simulink model "sldemo_bpcheck"  (Simulink 6.0)
settings: Solver=ode45  StartTime=0.0  StopTime=10.0  RelTol=1e-3
undefined symbols (not defined in the file or in its folder): membrane
libraries: simulink x9
settings Model: Creator=The MathWorks Inc.  LastModifiedBy=batserve  ExtModeAutoUpdateStatusClock=off
settings DataIOCC: SignalLoggingName=sigsOut
settings OptimizationCC: BooleanDataType=off
settings DebuggingCC: CheckExecutionContextPreStartOutputMsg=on  CheckExecutionContextRuntimeOutputMsg=on  SolverPrmCheckMsg=none
settings HardwareCC: TargetUnknown=on

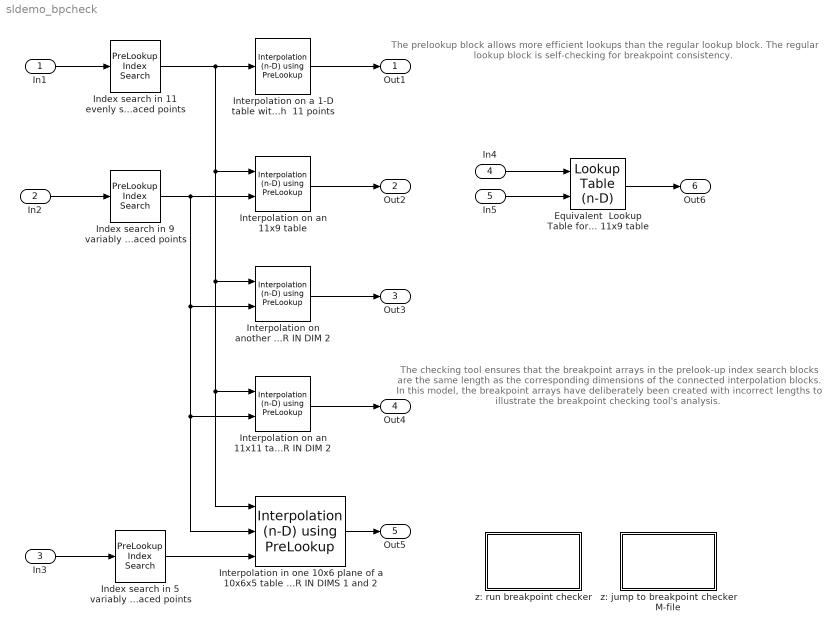
== system sldemo_bpcheck ==
  note: The checking tool ensures that
      | the breakpoint arrays in the
      | prelook-up index search blocks
      | are the same length as the
      | corresponding dimensions of the
      | connected interpolation blocks.
      |
      | In this model, the breakpoint arrays
      | have deliberately been created with
      |  incorrect lengths to illustrate the
      | breakpoint checking tool's analysis.
  note: The prelookup block allows  more
      | efficient lookups than the regular lookup
      | block.  The regular lookup block is
      | self-checking for breakpoint consistency.
  In1 : Inport  Port=1  LatchInput=off
  In2 : Inport  Port=2  LatchInput=off
  In3 : Inport  Port=3  LatchInput=off
  In4 : Inport  Port=4  LatchInput=off
  In5 : Inport  Port=5  LatchInput=off
  Equivalent  Lookup Table for Interpolation on an 11x9 table : simulink/Lookup Tables/Lookup Table (n-D)  numDimsPopupSelect=2  bp1=[0:10:100]  bp2=[ 0.5, 1, 3, 5, 15, 45, 95, 96, 97 ]  bp3=[1:3]  bp4=[1:3]  bpcell={ [1:3], [1:3] }  explicitNumDims=2  searchMode=Binary Search  cacheBpFlag=off  vectorInputFlag=off  tableData=reshape([1:99], [11,9])  interpMethod=Linear  extrapMethod=Linear  rangeErrorMode=None
  Index search in 11 evenly spaced points : simulink/Lookup Tables/PreLookup Index Search  bpData=[0:10:100]  searchMode=Evenly Spaced Points  cacheBpFlag=off  outputFlag=off  IndexDataType=uint32  extrapMode=Linear Extrapolation  rangeErrorMode=None
  Index search in 5 variably spaced points : simulink/Lookup Tables/PreLookup Index Search  bpData=[-100, 125, 150, 200, 500]  searchMode=Linear Search  cacheBpFlag=on  outputFlag=on  IndexDataType=uint32  extrapMode=Clip to Range  rangeErrorMode=Warning
  Index search in 9 variably spaced points : simulink/Lookup Tables/PreLookup Index Search  bpData=[ 0.5, 1, 3, 5, 15, 45, 95, 96, 97 ]  searchMode=Binary Search  cacheBpFlag=on  outputFlag=off  IndexDataType=uint32  extrapMode=Linear Extrapolation  rangeErrorMode=None
  Interpolation in one 10x6 plane of a 10x6x5 table ERROR IN DIMS 1 and 2 : simulink/Lookup Tables/Interpolation (n-D) using PreLookup  numDimsPopupSelect=3  explicitNumDims=2  table=reshape([1:300], [10,6,5])  interpMethod=Linear  extrapMethod=None - Clip  rangeErrorMode=None  NumSelectionDims=1
  Interpolation on a 1-D table with  11 points : simulink/Lookup Tables/Interpolation (n-D) using PreLookup  numDimsPopupSelect=1  explicitNumDims=2  table=[1:11].*[1:11]  interpMethod=Linear  extrapMethod=None - Clip  rangeErrorMode=None  NumSelectionDims=0
  Interpolation on an 11x11 table ERROR IN DIM 2 : simulink/Lookup Tables/Interpolation (n-D) using PreLookup  numDimsPopupSelect=2  explicitNumDims=2  table=sqrt([0:10]'*[0:10])  interpMethod=Linear  extrapMethod=Linear  rangeErrorMode=None  NumSelectionDims=0
  Interpolation on an 11x9 table : simulink/Lookup Tables/Interpolation (n-D) using PreLookup  numDimsPopupSelect=2  explicitNumDims=2  table=reshape([1:99], [11,9])  interpMethod=Linear  extrapMethod=None - Clip  rangeErrorMode=None  NumSelectionDims=0
  Interpolation on another 11x11 table ERROR IN DIM 2 : simulink/Lookup Tables/Interpolation (n-D) using PreLookup  numDimsPopupSelect=2  explicitNumDims=2  table=membrane(1,5,9,9)  interpMethod=Linear  extrapMethod=Linear  rangeErrorMode=None  NumSelectionDims=0
  z: jump to breakpoint checker M-file : Subsystem  PropExecContextAcrossSSBoundary=on
      settings: OpenFcn=edit slcheckprelookups.m
      mask Type: Demo
      mask Display: disp('View\nBreakpoint\nChecker')
  z: run breakpoint checker : Subsystem  PropExecContextAcrossSSBoundary=on
      settings: OpenFcn=evalin('base','preblks = slcheckprelookups(''sldemo_bpcheck''), commandwindow')
      mask Type: Demo
      mask Display: disp('Run\nBreakpoint\nChecker')
  Out1 : Outport
  Out2 : Outport  Port=2
  Out3 : Outport  Port=3
  Out4 : Outport  Port=4
  Out5 : Outport  Port=5
  Out6 : Outport  Port=6
  wires:
  Index search in 11 evenly spaced points/1 -> Interpolation in one 10x6 plane of a 10x6x5 table ERROR IN DIMS 1 and 2/1, Interpolation on an 11x11 table ERROR IN DIM 2/1, Interpolation on another 11x11 table ERROR IN DIM 2/1, Interpolation on an 11x9 table/1, Interpolation on a 1-D table with  11 points/1
  In1/1 -> Index search in 11 evenly spaced points/1
  In2/1 -> Index search in 9 variably spaced points/1
  Index search in 9 variably spaced points/1 -> Interpolation in one 10x6 plane of a 10x6x5 table ERROR IN DIMS 1 and 2/2, Interpolation on an 11x11 table ERROR IN DIM 2/2, Interpolation on another 11x11 table ERROR IN DIM 2/2, Interpolation on an 11x9 table/2
  In3/1 -> Index search in 5 variably spaced points/1
  Index search in 5 variably spaced points/1 -> Interpolation in one 10x6 plane of a 10x6x5 table ERROR IN DIMS 1 and 2/3
  Interpolation on an 11x9 table/1 -> Out2/1
  Interpolation on another 11x11 table ERROR IN DIM 2/1 -> Out3/1
  Interpolation in one 10x6 plane of a 10x6x5 table ERROR IN DIMS 1 and 2/1 -> Out5/1
  Interpolation on a 1-D table with  11 points/1 -> Out1/1
  Interpolation on an 11x11 table ERROR IN DIM 2/1 -> Out4/1
  In4/1 -> Equivalent  Lookup Table for Interpolation on an 11x9 table/1
  In5/1 -> Equivalent  Lookup Table for Interpolation on an 11x9 table/2
  Equivalent  Lookup Table for Interpolation on an 11x9 table/1 -> Out6/1

== system sldemo_bpcheck/z: jump to breakpoint checker M-file ==
  note: This block intentionally has no contents.

== system sldemo_bpcheck/z: run breakpoint checker ==
  note: This block intentionally has no contents.
